simulink model "rlVarTh_func_withController"  (R2020b)
settings: Solver=ode23t  StartTime=0.0  StopTime=Tf  RelTol=1e-2
model workspace: external: MAT-File C:\PhD\Variable Threshold\demo_rl.mat (data not in the file)
values from neighbouring files (symbols this model uses):
  Tf = 15    [main_rl_func_modified.m]
  Ts = 0.1    [main_rl_func_modified.m]
  whichAg_sim = whichAg_sim*5    (= 30)    [main_rl_func_modified.m]
undefined symbols (not defined in the file or in its folder): s
libraries: rllib x3, simulink x2
settings Model: Creator=The MathWorks, Inc.  LastModifiedBy=LENOVO

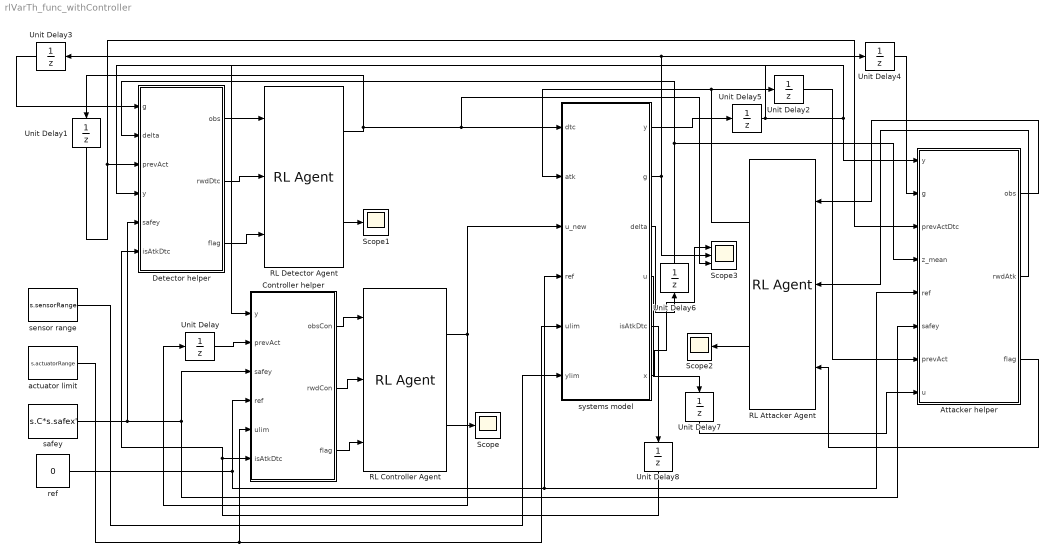
== system rlVarTh_func_withController ==
  Attacker helper : Subsystem
  Controller helper : Subsystem
  Detector helper : Subsystem
  RL Attacker Agent : rllib/RL Agent  Agent=agentAtk  ProvideReward=on  ProvideIsDone=on  ProvideCumRwd=on  TreatAsDirectFeedthrough=on  CollectLoggedSignals=on  CollectModelStates=on
  RL Controller Agent : rllib/RL Agent  Agent=agentCon  ProvideReward=on  ProvideIsDone=on  ProvideCumRwd=on  TreatAsDirectFeedthrough=on  CollectLoggedSignals=on  CollectModelStates=on
  RL Detector Agent : rllib/RL Agent  Agent=agentDtc  ProvideReward=on  ProvideIsDone=on  ProvideCumRwd=on  TreatAsDirectFeedthrough=on  CollectLoggedSignals=on  CollectModelStates=on
  Scope : Scope
  Scope1 : Scope
  Scope2 : Scope
  Scope3 : Scope  NumInputPorts=3
  Unit Delay{,1..8} (9 alike) : UnitDelay  SampleTime=-1  HasFrameUpgradeWarning=on
  actuator limit : Constant  Value=s.actuatorRange
  ref : Constant  Value=0
  safey : Constant  Value=s.C*s.safex'
  sensor range : Constant  Value=s.sensorRange
  systems model : Subsystem
  wires:
  Unit Delay5/1 -> Detector helper/4(y), Attacker helper/1(y), Controller helper/1(y)
  ref/1 -> systems model/4(ref), Attacker helper/5(ref), Controller helper/4(ref)
  safey/1 -> Detector helper/5(safey), Controller helper/3(safey), Attacker helper/6(safey)
  Unit Delay6/1 -> Detector helper/2(delta), Attacker helper/4(z_mean)
  Attacker helper/1(obs) -> RL Attacker Agent/1
  systems model/3(delta) -> Unit Delay6/1
  Unit Delay3/1 -> Detector helper/1(g)
  Controller helper/3(flag) -> RL Controller Agent/3
  Unit Delay1/1 -> Detector helper/3(prevAct), Attacker helper/3(prevActDtc)
  Controller helper/1(obsCon) -> RL Controller Agent/1
  Detector helper/2(rwdDtc) -> RL Detector Agent/2
  Unit Delay4/1 -> Attacker helper/2(g)
  Unit Delay/1 -> Controller helper/2(prevAct)
  Controller helper/2(rwdCon) -> RL Controller Agent/2
  Attacker helper/2(rwdAtk) -> RL Attacker Agent/2
  Attacker helper/3(flag) -> RL Attacker Agent/3
  sensor range/1 -> systems model/6(ylim)
  actuator limit/1 -> Controller helper/5(ulim), systems model/5(ulim)
  RL Controller Agent/1 -> systems model/3(u_new), Unit Delay/1
  Unit Delay2/1 -> Attacker helper/7(prevAct)
  Detector helper/3(flag) -> RL Detector Agent/3
  RL Attacker Agent/1 -> systems model/2(atk), Unit Delay2/1
  systems model/2(g) -> Scope3/2, Unit Delay4/1, Unit Delay3/1
  RL Detector Agent/1 -> Scope3/3, systems model/1(dtc), Unit Delay1/1
  RL Detector Agent/2 -> Scope1/1
  RL Attacker Agent/2 -> Scope2/1
  Detector helper/1(obs) -> RL Detector Agent/1
  RL Controller Agent/2 -> Scope/1
  systems model/1(y) -> Unit Delay5/1
  systems model/4(u) -> Unit Delay7/1
  Unit Delay7/1 -> Attacker helper/8(u)
  systems model/5(isAtkDtc) -> Unit Delay8/1
  Unit Delay8/1 -> Detector helper/6(isAtkDtc), Controller helper/6(isAtkDtc)
  systems model/6(x) -> Scope3/1

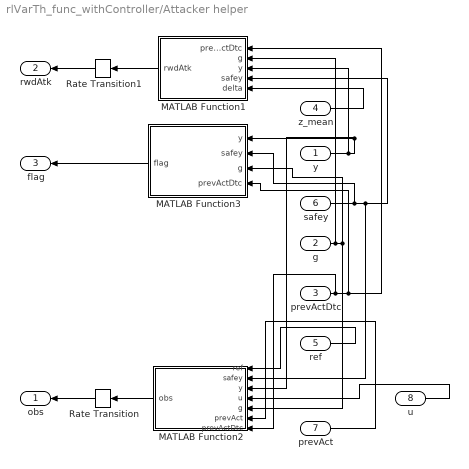
== system rlVarTh_func_withController/Attacker helper ==
  y : Inport
  g : Inport  Port=2
  prevActDtc : Inport  Port=3
  z_mean : Inport  Port=4
  ref : Inport  Port=5
  safey : Inport  Port=6
  prevAct : Inport  Port=7
  u : Inport  Port=8
  MATLAB Function1 : MATLAB Function  TreatAsAtomicUnit=on
  MATLAB Function2 : MATLAB Function  TreatAsAtomicUnit=on
  MATLAB Function3 : MATLAB Function  TreatAsAtomicUnit=on
  Rate Transition : RateTransition
  Rate Transition1 : RateTransition
  obs : Outport
  rwdAtk : Outport  Port=2
  flag : Outport  Port=3
  wires:
  Rate Transition1/1 -> rwdAtk/1
  MATLAB Function2/1(obs) -> Rate Transition/1
  Rate Transition/1 -> obs/1
  safey/1 -> MATLAB Function1/4(safey), MATLAB Function2/2(safey), MATLAB Function3/2(safey)
  MATLAB Function1/1(rwdAtk) -> Rate Transition1/1
  ref/1 -> MATLAB Function2/1(ref)
  z_mean/1 -> MATLAB Function1/5(delta)
  prevAct/1 -> MATLAB Function2/6(prevAct)
  g/1 -> MATLAB Function3/3(g), MATLAB Function2/5(g), MATLAB Function1/2(g)
  y/1 -> MATLAB Function2/3(y), MATLAB Function3/1(y), MATLAB Function1/3(y)
  prevActDtc/1 -> MATLAB Function3/4(prevActDtc), MATLAB Function1/1(prevActDtc), MATLAB Function2/7(prevActDtc)
  u/1 -> MATLAB Function2/4(u)
  MATLAB Function3/1(flag) -> flag/1

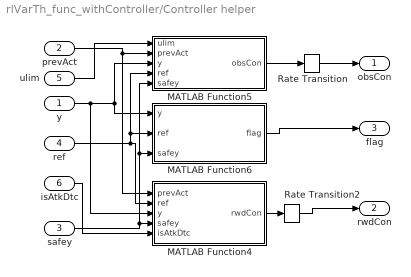
== system rlVarTh_func_withController/Controller helper ==
  y : Inport
  prevAct : Inport  Port=2
  safey : Inport  Port=3
  ref : Inport  Port=4
  ulim : Inport  Port=5
  isAtkDtc : Inport  Port=6
  MATLAB Function4 : MATLAB Function  TreatAsAtomicUnit=on
  MATLAB Function5 : MATLAB Function  TreatAsAtomicUnit=on
  MATLAB Function6 : MATLAB Function  TreatAsAtomicUnit=on
  Rate Transition : RateTransition
  Rate Transition2 : RateTransition
  obsCon : Outport
  rwdCon : Outport  Port=2
  flag : Outport  Port=3
  wires:
  ref/1 -> MATLAB Function6/2(ref), MATLAB Function5/4(ref), MATLAB Function4/2(ref)
  safey/1 -> MATLAB Function5/5(safey), MATLAB Function6/3(safey), MATLAB Function4/4(safey)
  MATLAB Function4/1(rwdCon) -> Rate Transition2/1
  MATLAB Function5/1(obsCon) -> Rate Transition/1
  y/1 -> MATLAB Function6/1(y), MATLAB Function5/3(y), MATLAB Function4/3(y)
  prevAct/1 -> MATLAB Function4/1(prevAct), MATLAB Function5/2(prevAct)
  Rate Transition/1 -> obsCon/1
  MATLAB Function6/1(flag) -> flag/1
  ulim/1 -> MATLAB Function5/1(ulim)
  Rate Transition2/1 -> rwdCon/1
  isAtkDtc/1 -> MATLAB Function4/5(isAtkDtc)

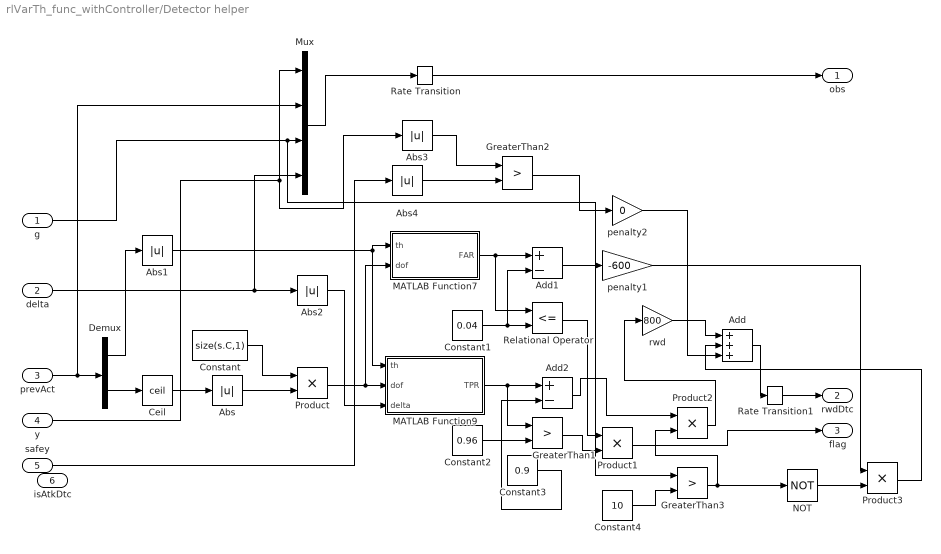
== system rlVarTh_func_withController/Detector helper ==
  g : Inport
  delta : Inport  Port=2
  prevAct : Inport  Port=3
  y : Inport  Port=4
  safey : Inport  Port=5
  isAtkDtc : Inport  Port=6
  Abs{,1..4} (5 alike) : Abs
  Add : Sum  Inputs=+++
  Add1 : Sum  Inputs=+-
  Add2 : Sum  Inputs=+-
  Ceil : Rounding  Operator=ceil
  Constant : Constant  Value=size(s.C,1)  SampleTime=Ts
  Constant1 : Constant  Value=0.04  SampleTime=Ts
  Constant2 : Constant  Value=0.96  SampleTime=Ts
  Constant3 : Constant  Value=0.9  SampleTime=Ts
  Constant4 : Constant  Value=10  SampleTime=Ts
  Demux : Demux  Outputs=2
  GreaterThan1 : RelationalOperator  Operator=>  OutDataTypeStr=boolean  RndMeth=Simplest
  GreaterThan2 : RelationalOperator  Operator=>  OutDataTypeStr=boolean  RndMeth=Simplest
  GreaterThan3 : RelationalOperator  Operator=>  OutDataTypeStr=boolean  RndMeth=Simplest
  MATLAB Function7 : MATLAB Function  TreatAsAtomicUnit=on
  MATLAB Function9 : MATLAB Function  TreatAsAtomicUnit=on
  Mux : Mux
  NOT : Logic  Operator=NOT  IconShape=distinctive  AllPortsSameDT=off  OutDataTypeStr=boolean
  Product{,1..3} (4 alike) : Product
  Rate Transition : RateTransition
  Rate Transition1 : RateTransition
  Relational Operator : RelationalOperator  Operator=<=  OutDataTypeStr=boolean  RndMeth=Simplest
  penalty1 : Gain  Gain=-600
  penalty2 : Gain  Gain=0
  rwd : Gain  Gain=800
  obs : Outport
  rwdDtc : Outport  Port=2
  flag : Outport  Port=3
  wires:
  Demux/2 -> Ceil/1
  Constant2/1 -> GreaterThan1/2
  GreaterThan1/1 -> Product1/2
  Relational Operator/1 -> Product1/1
  MATLAB Function9/1(TPR) -> Add2/1, GreaterThan1/1
  Add/1 -> Rate Transition1/1
  Ceil/1 -> Abs/1
  penalty2/1 -> Add/3
  rwd/1 -> Add/1
  Add1/1 -> penalty1/1
  Rate Transition/1 -> obs/1
  Abs/1 -> Product/2
  Demux/1 -> Abs1/1
  MATLAB Function7/1(FAR) -> Relational Operator/1, Add1/1
  Constant1/1 -> Add1/2, Relational Operator/2
  Rate Transition1/1 -> rwdDtc/1
  Mux/1 -> Rate Transition/1
  Constant/1 -> Product/1
  Product/1 -> MATLAB Function9/2(dof), MATLAB Function7/2(dof)
  g/1 -> GreaterThan3/1, Mux/3
  delta/1 -> Mux/4, Abs2/1
  prevAct/1 -> Demux/1, Mux/2
  Abs1/1 -> MATLAB Function7/1(th), MATLAB Function9/1(th)
  y/1 -> Mux/1, Abs3/1
  GreaterThan2/1 -> penalty2/1
  Abs3/1 -> GreaterThan2/1
  Abs4/1 -> GreaterThan2/2
  safey/1 -> Abs4/1
  Product1/1 -> flag/1
  Constant3/1 -> Add2/2
  Add2/1 -> Product2/1
  Constant4/1 -> GreaterThan3/2
  Abs2/1 -> MATLAB Function9/3(delta)
  GreaterThan3/1 -> NOT/1, Product2/2
  Product2/1 -> rwd/1
  NOT/1 -> Product3/2
  penalty1/1 -> Product3/1
  Product3/1 -> Add/2

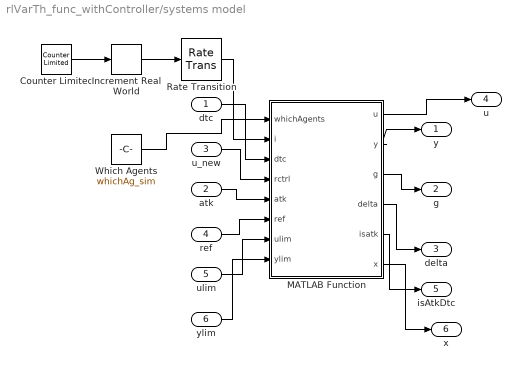
== system rlVarTh_func_withController/systems model ==
  dtc : Inport
  atk : Inport  Port=2
  u_new : Inport  Port=3
  ref : Inport  Port=4
  ulim : Inport  Port=5
  ylim : Inport  Port=6
  Counter Limited : simulink/Sources/Counter Limited  uplimit=Tf/Ts-2  tsamp=Ts
  Increment Real World : simulink/Additional Math & Discrete/Additional Math: Increment - Decrement/Increment Real World
      settings: SourceProductBaseCode=SL
  MATLAB Function : MATLAB Function  TreatAsAtomicUnit=on
  Rate Transition : RateTransition
  Which Agents : Constant  Value=whichAg_sim  SampleTime=Ts
  y : Outport
  g : Outport  Port=2
  delta : Outport  Port=3
  u : Outport  Port=4
  isAtkDtc : Outport  Port=5
  x : Outport  Port=6
  wires:
  ref/1 -> MATLAB Function/6(ref)
  ylim/1 -> MATLAB Function/8(ylim)
  MATLAB Function/4(delta) -> delta/1
  atk/1 -> MATLAB Function/5(atk)
  Increment Real World/1 -> Rate Transition/1
  Rate Transition/1 -> MATLAB Function/2(i)
  MATLAB Function/3(g) -> g/1
  ulim/1 -> MATLAB Function/7(ulim)
  dtc/1 -> MATLAB Function/3(dtc)
  Counter Limited/1 -> Increment Real World/1
  MATLAB Function/2(y) -> y/1
  u_new/1 -> MATLAB Function/4(rctrl)
  MATLAB Function/1(u) -> u/1
  Which Agents/1 -> MATLAB Function/1(whichAgents)
  MATLAB Function/5(isatk) -> isAtkDtc/1
  MATLAB Function/6(x) -> x/1

== matlab function rlVarTh_func_withController/Controller helper/MATLAB Function6 ==
  data: y input; ref input; flag output; safey input
function flag = stop(y,ref,safey)
flag= 0;
% flag = abs((y-ref)/ref) <= 0.25;

== matlab function rlVarTh_func_withController/Detector helper/MATLAB Function7 ==
  data: FAR output; th input; dof input
function FAR  = calcFAR(th,dof)
%    format long g;
   FAR = chi2cdf(th,dof,'upper')

== matlab function rlVarTh_func_withController/Detector helper/MATLAB Function9 ==
  data: th input; dof input; TPR output; delta input
function TPR  = calcTPR(th,dof,delta)
%    format long g;
   TPR = ncx2cdf(th,dof,delta,'upper')
end

== matlab function rlVarTh_func_withController/Attacker helper/MATLAB Function1 ==
  data: rwdAtk output; prevActDtc input; g input; y input; safey input; delta input
function rwdAtk  = rwrdAtk(prevActDtc,g,y,safey,delta)
%    format long g;
   th = abs(prevActDtc(1))
   tau = max(1,ceil(prevActDtc(2,1)))
   dof = size(y,1)*(tau)
   FAR = chi2cdf(th,dof,'upper')
   TPR = ncx2cdf(th,dof,abs(delta),'upper')
%    rwdAtk = FAR/TPR + 50*(g<th)+ 100*(y-ref)^2;
%             50*(FAR-0.05)-40*TPR + 50*(g<th)+ 100*(abs(y)-abs(safey))
% % rwdAtk = 50*(1-FAR) -50*TPR + 100*(g<th & abs(y)>abs(safey))+ 100*(abs(y)-abs(safey))
% rwdAtk = 50*(-FAR) -50*TPR + 100*(g<th)*(abs(y)-abs(safey))+ 100*(g<th)*(abs(y)-0.3*abs(safey))


% rwdAtk = 50*(FAR) -50*TPR + 10000*(g<th)*(abs(y)-abs(safey))+ 10000*(g<th)*(abs(y)-0.3*abs(safey))

rwdAtk = 50*(FAR) -50*TPR + 10000*(g<th)*(abs(y)-0.3*abs(safey))

== matlab function rlVarTh_func_withController/systems model/MATLAB Function ==
  data: whichAgents input; u output; i input; y output; g output; delta output; dtc input; rctrl input; atk input; ref input; ulim input; ylim input; s parameter; isatk output; x output
function [u,y,g,delta,isatk,x] = env(whichAgents,i,dtc,rctrl,atk,ref,ulim,ylim, s)
% function [y,g,z_mean]= envSys(atk,dtc,new_u,ref, s)
%% SYS_ENV Summary of this function goes here

%%%%%%%%%%%%%%%%%%%%%%%%%%%=====FDI Attack=========%%%%%%%%%%%%%%%%%%%%%
%========================== obtained from code ======================%
% x1_0=-15.0;
% x2_0=16.6096079397;
% fdi_u=[ 35.99313719  71.98627437  58.33575204  41.29588025   0.   0.         -31.21892088  -5.09118639   0.           0.  -0.41831677   0.           0.           0.           0.   0. ];
% fdi_y=[15.01515367 13.48175215 11.26355514 10.30553807  8.22658704  4.85366237  3.61911687  2.21566942  1.21608204  0.53164255  0.1748743   0.  0.          0.          0.          0. ];
%======================================================================%

% ay=  [fdi_y,zeros(1,time-size(fdi_y,2))];
% au = [fdi_u,zeros(1,time-size(fdi_u,2))];

%%%%%%%%%%%%%%%%%%%%%%%%%%=====System Simulation======%%%%%%%%%%%%%%%%%%

%====================Chi Squared Test =================
% tau = 1; % Detection window % new: let's check for every iteration now
%======================================================
% stateProg(esp_env,i,dtc(2),dtc(1),new_u,atk(1),atk(2))

% 2 for attcker agent
if ~rem(whichAgents,2)
    au= atk(1);
    ay= atk(2);
    disp("with attacker agent")
else
    au=0;
    ay=0;
end
% 3 for controller agent
if ~rem(whichAgents,3)
    u_new= rctrl;
    disp("with controller agent")
else
    u_new = 0;
end
% 5 for detector agent
if ~rem(whichAgents,5)
    th= abs(dtc(1));
    dtc_windw= max(1,(ceil(dtc(2))));
    disp("with detector agent")
else
    th=4.35;%esp
    dtc_windw=1;
end
% coder.extrinsic('evalin','assignin');
% evalin
%  for i = 1:esp_env.Ts:esp_env.Tf
% th= abs(dtc(1));
% dtc_windw= max(1,(ceil(dtc(2))));
% u_new= rctrl;
% au= atk(1);
% ay= atk(2);
    s.x_act(:,1)
            s.t(i+1)=s.t(i)+s.Ts;
            s.a_u(:,i+1)=au;
            s.a_y(:,i+1)=ay;
            s.x_act(:,i+1) = s.A*s.x_act(:,i)+s.B*s.uatk(:,i)+s.proc_noise(i);
%             s.xatk(i)= s.A*s.x_act(i)+s.B*s.u_act(i);
            s.xhat(:,i+1) = s.A*s.xhat(:,i) + s.B*s.u_act(:,i) + s.L*s.z(:,i);
            s.est_err(:,i+1)= s.x_act(:,i+1)-s.xhat(:,i+1);
            s.u_act(:,i+1)= max(-ulim,min(ulim,s.K*s.xhat(:,i+1)));
            s.uatk(:,i+1)= max(-ulim,min(ulim,s.u_act(:,i+1)+s.a_u(:,i+1)));
            s.y_act(:,i+1)= max(-ylim,min(ylim,s.C*s.x_act(:,i+1))+s.meas_noise(i));
            s.yatk(:,i+1)= max(-ylim,min(ylim,s.y_act(:,i+1)+s.a_y(:,i+1)));
            s.z(:,i+1)= s.yatk(:,i+1)-s.C*s.xhat(:,i+1);
            s.z_mean(:,i+1)= mean(s.z');
            s.z_var(:,i+1) = var(s.z');
%             s.chi_tst(i+1)= s.z(:,i+1)'*inv(s.z_var(:,i+1))*s.z(:,i+1);
            s.chi_tst(i+1)= s.z(:,i+1)'*(1/0.05)*s.z(:,i+1);
%             s.chi_tst(i+1)= s.z(:,i+1)'*inv(cov(s.z'))*s.z(:,i+1);
            
             if ~isfinite(s.chi_tst(i+1))
                    s.chi_tst(i+1)= 0;
             end
            s.threshold(i+1)= th;
            s.tau(i+1)= dtc_windw;
            s.g(i+1) = 0;       
            s.non_cent(i+1)= 0;
%             if i-tau+1 > 0                  % Calculate detector window starting index
%                 srt = i-tau+1;              % tau is the detector window length
%             else
%                 srt = 1;
%             end
%% Chi square test and non centrality calculation
            for k = max(1,i-s.tau(i+1)+1):i
                s.g(i+1) = s.g(i+1) + s.chi_tst(k+1);  % Calculate gk (chi2 test)
                del= s.z_mean(:,k+1)'*inv(s.z_var(k+1))*s.z_mean(:,k+1);
%                 del= s.z_mean(:,k+1)'*inv(cov(s.z'))*s.z_mean(:,k+1);
                if ~isfinite(del)
                    s.non_cent(i+1)= s.non_cent(i+1) + 0;
                else
                    s.non_cent(i+1)= s.non_cent(i+1) + del;
                end
            end
            
%% to start the RL based controller
            if ((abs(s.yatk(i+1))>abs(s.C*s.safex'))) || (s.g(i+1) > s.threshold(i+1))
                s.u_act(:,i+1) = max(-ulim,min(ulim,u_new));
                s.uatk(:,i+1)= max(-ulim,min(ulim,s.u_act(:,i+1)+s.a_u(:,i+1)));
                isatk=1;
                disp("detected");
%                 plot(s.yatk);
%                 hold on;
%                 plot(s.z');
%                 hold on;
%                 plot(s.g');
%                 hold on;
%                 plot(s.threshold');
%                 hold on;
%                 plot((s.safex*ones(size(s.A,1),size(s.t,2)))');
%                 hold on;
%                 plot((s.safex*ones(size(s.A,1),size(s.t,2)))');
%                 hold off;
            else
                isatk=0;
            end
    disp("iteration: "+i)     
    dof=s.tau(i+1)*size(s.C,1)     
    th=s.threshold(i+1)     
    FAR = chi2cdf(th,dof,'upper');     
    TPR = ncx2cdf(th,dof,s.non_cent(i+1),'upper')     
    avgtpr=s.avgtpr+TPR     
    avgfar=s.avgfar+FAR     
    s.avgfar=avgfar;     
    s.avgtpr=avgtpr;     
    zm=s.z_mean(i+1)     
    zv=s.z_var(i+1)     
    ct=s.chi_tst(i+1)     
    g= s.g(i+1)     
    y=s.yatk(:,i+1)     
    u=s.uatk(:,i+1)     
    delta = s.non_cent(i+1)     
    fdi=[ay; au]     
    x= s.x_act(:,i+1)
   
   
end

== matlab function rlVarTh_func_withController/Attacker helper/MATLAB Function2 ==
  data: obs output; ref input; safey input; y input; u input; g input; prevAct input; prevActDtc input
function obs = obsAtk(ref,safey,y,u,g,prevAct,prevActDtc)
%     format long g;
    ay= prevAct(1,1);
    au= prevAct(2,1);
    obs= [ref;y-ay;u-au;g;safey;prevAct;prevActDtc];

== matlab function rlVarTh_func_withController/Attacker helper/MATLAB Function3 ==
  data: y input; flag output; safey input; g input; prevActDtc input
function flag  = stop(y,safey, g, prevActDtc)
%     format long g;
    th = abs(prevActDtc(1));
%     flag = y > safey & g <= th;
flag=0;

== matlab function rlVarTh_func_withController/Controller helper/MATLAB Function4 ==
  data: rwdCon output; prevAct input; ref input; y input; safey input; isAtkDtc input
function rwdCon  = rwrdCon(prevAct,ref,y,safey,isAtkDtc)
%     format long g;
    u=prevAct;
%     ay=atk(2);
    %% safer : 0.5* safey
%     rwdCon = 350*(abs((y-ref)/ref) <= 0.30)-20*(prevAct)^2-100*(abs(y) > safey)-50
% rwdCon = isAtkDtc*(-100*(y-0.4*safey)^2-200*(abs(y)-abs(safey)))%-20*u^2
rwdCon = isAtkDtc*(-10000*(y-0.3*safey)^2)%-20*u^2

== matlab function rlVarTh_func_withController/Controller helper/MATLAB Function5 ==
  data: ulim input; obsCon output; prevAct input; y input; ref input; safey input
function obsCon = obsCon(ulim,prevAct,y,ref,safey)
   
    obsCon=[ulim;prevAct;y;ref;safey];
